simulink model "image_analysis_color"  (Simulink 7.6)
settings: Solver=FixedStepDiscrete  StartTime=0.0  StopTime=0  RelTol=1e-3
undefined symbols (not defined in the file or in its folder): Iter_Segment_Thresh, jet, Rec, SDTV
libraries: vipsnks x16, vipconversions x11, vipanalysis x4, vipgeotforms x3, viptransforms x2, vipsrcs x1, viptextngfix x1
settings Model: Creator=Administrator  LastModifiedBy=Administrator

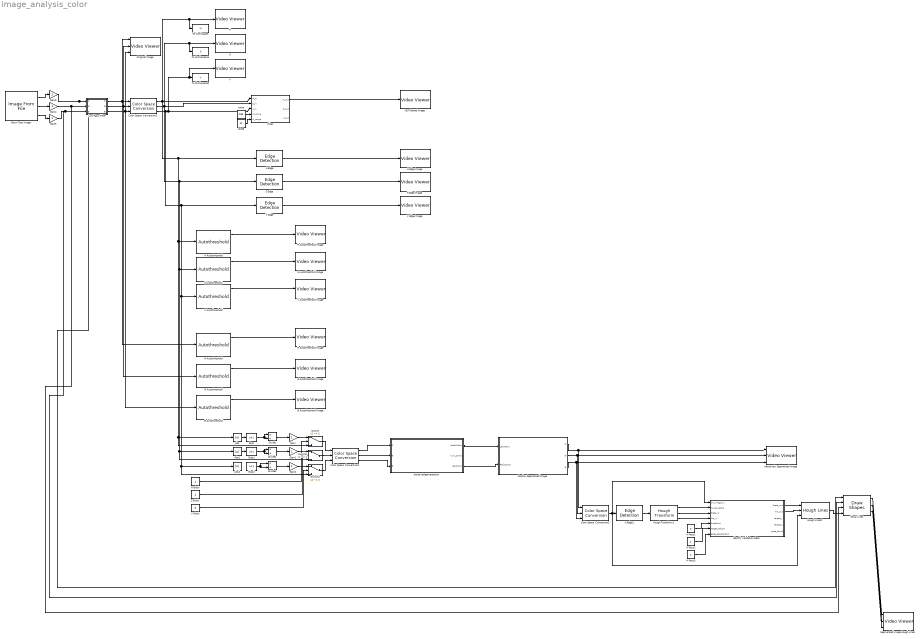
== system image_analysis_color ==
  Abs : Abs
  Abs1 : Abs
  Abs2 : Abs
  B Autothreshold : vipconversions/Autothreshold  DialogController=vipDDGCreate  DialogControllerArgs=DataTag0  operator=>  threshOut=on  effMetricOut=on  userDefinedRange=off  umin=0  umax=255  outOfRngOpt=Warn and saturate  scaleThreshold=off  scaleFactor=1  P1Mode=Specify word length  P1WordLength=32  P1FracLength=30  P2Mode=Specify word length  P2WordLength=32  P2FracLength=22  P3Mode=Specify word length  P3WordLength=32  P3FracLength=14  P4Mode=Binary point scaling  P4WordLength=32  P4FracLength=15  Q1Mode=Specify word length  Q1WordLength=32  Q1FracLength=16  EMMode=Specify word length  EMWordLength=16  EMFracLength=14  roundingMode=Floor  overflowMode=off
  B Autothreshold Image : vipsnks/Video Viewer  DialogControllerArgs=DataTag2  inputType=Obsolete7b  imagePorts=One multidimensional signal  useColorMap=off  colormapValue=jet(256)  specRange=off  minInputVal=0  maxInputVal=255  FigPos=[805 664 208 170]  AxisZoom=on  trueSizedOnce=off  OpenAtMdlStart=on
  Bias : Bias  Bias=1
  Bias1 : Bias  Bias=1
  Bias2 : Bias  Bias=1
  Color Space  Conversion1 : vipconversions/Color Space  Conversion  conversion=Obsolete  conversionActive=R'G'B' to HSV  wp_str=D65  rec=Rec. 601 (SDTV)  sys=1125/60/2:1  imagePorts=Separate color signals
  Color Space  Conversion2 : vipconversions/Color Space  Conversion  conversion=Obsolete  conversionActive=HSV to R'G'B'  wp_str=D65  rec=Rec. 601 (SDTV)  sys=1125/60/2:1  imagePorts=Separate color signals
  Color Space  Conversion3 : vipconversions/Color Space  Conversion  conversion=Obsolete  conversionActive=R'G'B' to intensity  wp_str=D65  rec=Rec. 601 (SDTV)  sys=1125/60/2:1  imagePorts=Separate color signals
  Display Segmented Image : Subsystem
      settings: UndoDeleteFcn=Stateflow.SLINSF.SimulinkMan.restorePreDeleteFcn  PreDeleteFcn=Stateflow.SLINSF.SimulinkMan.removePreDeleteFcn
  Divide : Product  Inputs=*/
  Divide1 : Product  Inputs=*/
  Divide2 : Product  Inputs=*/
  Down Test Image : vipsrcs/Image From File  Tag=vipblks_nd  DialogController=vipDDGCreate  DialogControllerArgs=DataTag3  SystemSampleTime=-1  FileName=C:\Documents and Settings\Administrator\My Documents\Academics\Summer 2011\Digital Image Correlation\Sample Pictures 5-24-11\sample1_small.JPG  imagePorts=Separate color signals  Ts=-1  ImageDataType=double  Signed=on  WordLength=16  sdImageDataType=uint(8)  FractionLengthMode=User-defined  FractionLength=15  OutPortLabels=R|G|B
  Draw Lines : viptextngfix/Draw Shapes  DialogController=vipDDGCreate  DialogControllerArgs=DataTag4  shape=Lines  fill=off  fillClrSource=Specify via dialog  display=User-specified value  intensity=200  color=[.8 .8 .8]  opacity=0.6  viewport=Entire image  antialiasing=off  inType=Obsolete  imagePorts=Separate color signals  prodOutputMode=Binary point scaling  prodOutputWordLength=32  prodOutputFracLength=14  memoryMode=Specify word length  memoryWordLength=16  memoryFracLength=15  roundingMode=Floor  overflowMode=off
  Filter : Stateflow chart  TreatAsAtomicUnit=on
  G Autothreshold : vipconversions/Autothreshold  DialogController=vipDDGCreate  DialogControllerArgs=DataTag5  operator=>  threshOut=on  effMetricOut=on  userDefinedRange=off  umin=0  umax=255  outOfRngOpt=Warn and saturate  scaleThreshold=off  scaleFactor=1  P1Mode=Specify word length  P1WordLength=32  P1FracLength=30  P2Mode=Specify word length  P2WordLength=32  P2FracLength=22  P3Mode=Specify word length  P3WordLength=32  P3FracLength=14  P4Mode=Binary point scaling  P4WordLength=32  P4FracLength=15  Q1Mode=Specify word length  Q1WordLength=32  Q1FracLength=16  EMMode=Specify word length  EMWordLength=16  EMFracLength=14  roundingMode=Floor  overflowMode=off
  G Autothreshold Image : vipsnks/Video Viewer  DialogControllerArgs=DataTag7  inputType=Obsolete7b  imagePorts=One multidimensional signal  useColorMap=off  colormapValue=jet(256)  specRange=off  minInputVal=0  maxInputVal=255  FigPos=[794 437 202 172]  AxisZoom=on  trueSizedOnce=off  OpenAtMdlStart=on
  Gain{,1..5} (6 alike) : Gain
  H : vipsnks/Video Viewer  DialogControllerArgs=DataTag9  inputType=Obsolete7b  imagePorts=One multidimensional signal  useColorMap=off  colormapValue=jet(256)  specRange=off  minInputVal=0  maxInputVal=255  FigPos=[177 241 253 152]  AxisZoom=on  trueSizedOnce=off  OpenAtMdlStart=on
  H Autothreshold : vipconversions/Autothreshold  DialogController=vipDDGCreate  DialogControllerArgs=DataTag10  operator=>  threshOut=on  effMetricOut=on  userDefinedRange=off  umin=0  umax=255  outOfRngOpt=Warn and saturate  scaleThreshold=off  scaleFactor=1  P1Mode=Specify word length  P1WordLength=32  P1FracLength=30  P2Mode=Specify word length  P2WordLength=32  P2FracLength=22  P3Mode=Specify word length  P3WordLength=32  P3FracLength=14  P4Mode=Binary point scaling  P4WordLength=32  P4FracLength=15  Q1Mode=Specify word length  Q1WordLength=32  Q1FracLength=16  EMMode=Specify word length  EMWordLength=16  EMFracLength=14  roundingMode=Floor  overflowMode=off
  H Autothreshold Image : vipsnks/Video Viewer  DialogControllerArgs=DataTag12  inputType=Obsolete7b  imagePorts=One multidimensional signal  useColorMap=off  colormapValue=jet(256)  specRange=off  minInputVal=0  maxInputVal=255  FigPos=[602 227 224 146]  AxisZoom=on  trueSizedOnce=off  OpenAtMdlStart=on
  H Block : Constant
  H Edge : vipanalysis/Edge Detection  DialogController=vipDDGCreate  DialogControllerArgs=DataTag13  method=Sobel  outputType=Binary image  userDefinedThreshold=off  thresholdSource=Specify via dialog  threshold=20  thresholdTuning=3  edgeThinning=on  threshold_canny=[0.25 0.60]  autoPercent=70  sigma=1  roundingMode=Floor  overflowMode=off
  H Edge Image : vipsnks/Video Viewer  DialogControllerArgs=DataTag15  inputType=Obsolete7b  imagePorts=One multidimensional signal  useColorMap=off  colormapValue=jet(256)  specRange=off  minInputVal=0  maxInputVal=255  FigPos=[390 221 222 140]  AxisZoom=on  trueSizedOnce=off  OpenAtMdlStart=on
  H Edge1 : vipanalysis/Edge Detection  DialogController=vipDDGCreate  DialogControllerArgs=DataTag16  method=Sobel  outputType=Binary image  userDefinedThreshold=off  thresholdSource=Specify via dialog  threshold=20  thresholdTuning=3  edgeThinning=on  threshold_canny=[0.25 0.60]  autoPercent=70  sigma=1  roundingMode=Floor  overflowMode=off
  H Pass1 : Constant  Value=0
  H Pass2 : Constant
  H Pass3 : Constant
  HS Filtered Image : vipsnks/Video Viewer  DialogControllerArgs=DataTag18  inputType=Obsolete7b  imagePorts=One multidimensional signal  useColorMap=off  colormapValue=jet(256)  specRange=off  minInputVal=0  maxInputVal=255  FigPos=[-38 479 226 177]  AxisZoom=on  trueSizedOnce=off  OpenAtMdlStart=on
  Hough Lines2 : viptransforms/Hough Lines  DialogController=vipDDGCreate  DialogControllerArgs=DataTag19  sineCompMethod=Trigonometric function  thetaRes=pi/180  firstCoeffMode=Specify word length  firstCoeffWordLength=16  firstCoeffFracLength=15  prodOutputMode=Binary point scaling  prodOutputWordLength=32  prodOutputFracLength=16  roundingMode=Nearest  overflowMode=on
  Hough Transform1 : viptransforms/Hough Transform  DialogController=vipDDGCreate  DialogControllerArgs=DataTag20  theta_res=pi/180  rho_res=1  out_theta_rho=on  outdtmode=double  firstCoeffMode=Binary point scaling  firstCoeffWordLength=16  firstCoeffFracLength=14  secondCoeffMode=Binary point scaling  secondCoeffWordLength=32  secondCoeffFracLength=16  outputMode=Binary point scaling  outputWordLength=16  outputFracLength=0  accumMode=Binary point scaling  accumWordLength=32  accumFracLength=20  prodOutputMode=Binary point scaling  prodOutputWordLength=32  prodOutputFracLength=20  memoryMode=Binary point scaling  memoryWordLength=32  memoryFracLength=16  roundingMode=Nearest  overflowMode=on
  Identify Validation Gate : Stateflow chart  TreatAsAtomicUnit=on  SystemSampleTime=[1/30 0]
  IterativeSegmentation : Subsystem
      settings: UndoDeleteFcn=Stateflow.SLINSF.SimulinkMan.restorePreDeleteFcn  PreDeleteFcn=Stateflow.SLINSF.SimulinkMan.removePreDeleteFcn
  Iteratively Segmented Image : vipsnks/Video Viewer  DialogControllerArgs=DataTag25  inputType=Obsolete7b  imagePorts=Separate color signals  useColorMap=off  colormapValue=jet(256)  specRange=off  minInputVal=0  maxInputVal=255  FigPos=[1060 242 237 156]  AxisZoom=on  trueSizedOnce=off  OpenAtMdlStart=on
  Low Pass Filter : Subsystem
  Original Image : vipsnks/Video Viewer  DialogControllerArgs=DataTag27  inputType=Obsolete7b  imagePorts=Separate color signals  useColorMap=off  colormapValue=jet(256)  specRange=off  minInputVal=0  maxInputVal=255  FigPos=[-27 258 221 180]  AxisZoom=on  trueSizedOnce=off  OpenAtMdlStart=on
  R Autothreshold : vipconversions/Autothreshold  DialogController=vipDDGCreate  DialogControllerArgs=DataTag28  operator=>  threshOut=on  effMetricOut=on  userDefinedRange=off  umin=0  umax=255  outOfRngOpt=Warn and saturate  scaleThreshold=off  scaleFactor=1  P1Mode=Specify word length  P1WordLength=32  P1FracLength=30  P2Mode=Specify word length  P2WordLength=32  P2FracLength=22  P3Mode=Specify word length  P3WordLength=32  P3FracLength=14  P4Mode=Binary point scaling  P4WordLength=32  P4FracLength=15  Q1Mode=Specify word length  Q1WordLength=32  Q1FracLength=16  EMMode=Specify word length  EMWordLength=16  EMFracLength=14  roundingMode=Floor  overflowMode=off
  R Autothreshold Image : vipsnks/Video Viewer  DialogControllerArgs=DataTag30  inputType=Obsolete7b  imagePorts=One multidimensional signal  useColorMap=off  colormapValue=jet(256)  specRange=off  minInputVal=0  maxInputVal=255  FigPos=[794 238 224 156]  AxisZoom=on  trueSizedOnce=off  OpenAtMdlStart=on
  S : vipsnks/Video Viewer  DialogControllerArgs=DataTag32  inputType=Obsolete7b  imagePorts=One multidimensional signal  useColorMap=off  colormapValue=jet(256)  specRange=off  minInputVal=0  maxInputVal=255  FigPos=[193 436 207 154]  AxisZoom=on  trueSizedOnce=off  OpenAtMdlStart=on
  S Autothreshold : vipconversions/Autothreshold  DialogController=vipDDGCreate  DialogControllerArgs=DataTag33  operator=>  threshOut=on  effMetricOut=on  userDefinedRange=off  umin=0  umax=255  outOfRngOpt=Warn and saturate  scaleThreshold=off  scaleFactor=1  P1Mode=Specify word length  P1WordLength=32  P1FracLength=30  P2Mode=Specify word length  P2WordLength=32  P2FracLength=22  P3Mode=Specify word length  P3WordLength=32  P3FracLength=14  P4Mode=Binary point scaling  P4WordLength=32  P4FracLength=15  Q1Mode=Specify word length  Q1WordLength=32  Q1FracLength=16  EMMode=Specify word length  EMWordLength=16  EMFracLength=14  roundingMode=Floor  overflowMode=off
  S Autothreshold Image : vipsnks/Video Viewer  DialogControllerArgs=DataTag35  inputType=Obsolete7b  imagePorts=One multidimensional signal  useColorMap=off  colormapValue=jet(256)  specRange=off  minInputVal=0  maxInputVal=255  FigPos=[572 439 254 167]  AxisZoom=on  trueSizedOnce=off  OpenAtMdlStart=on
  S Block : Constant
  S Edge : vipanalysis/Edge Detection  DialogController=vipDDGCreate  DialogControllerArgs=DataTag36  method=Sobel  outputType=Binary image  userDefinedThreshold=off  thresholdSource=Specify via dialog  threshold=20  thresholdTuning=3  edgeThinning=on  threshold_canny=[0.25 0.60]  autoPercent=70  sigma=1  roundingMode=Floor  overflowMode=off
  S Edge Image : vipsnks/Video Viewer  DialogControllerArgs=DataTag38  inputType=Obsolete7b  imagePorts=One multidimensional signal  useColorMap=off  colormapValue=jet(256)  specRange=off  minInputVal=0  maxInputVal=255  FigPos=[396 426 193 132]  AxisZoom=on  trueSizedOnce=off  OpenAtMdlStart=on
  Segmented Image Hough Lines : vipsnks/Video Viewer  DialogControllerArgs=DataTag40  inputType=Obsolete7b  imagePorts=Separate color signals  useColorMap=off  colormapValue=jet(256)  specRange=off  minInputVal=0  maxInputVal=255  FigPos=[1009 491 272 162]  AxisZoom=on  trueSizedOnce=off  OpenAtMdlStart=on
  Switch : Switch  Criteria=u2 ~= 0
  Switch1 : Switch  Criteria=u2 ~= 0
  Switch2 : Switch  Criteria=u2 ~= 0
  To Workspace : ToWorkspace  VariableName=H  SampleTime=-1  SaveFormat=Array
  To Workspace1 : ToWorkspace  VariableName=S  SampleTime=-1  SaveFormat=Array
  To Workspace2 : ToWorkspace  VariableName=V  SampleTime=-1  SaveFormat=Array
  V : vipsnks/Video Viewer  DialogControllerArgs=DataTag42  inputType=Obsolete7b  imagePorts=One multidimensional signal  useColorMap=off  colormapValue=jet(256)  specRange=off  minInputVal=0  maxInputVal=255  FigPos=[202 649 196 150]  AxisZoom=on  trueSizedOnce=off  OpenAtMdlStart=on
  V Autothreshold : vipconversions/Autothreshold  DialogController=vipDDGCreate  DialogControllerArgs=DataTag43  operator=>  threshOut=on  effMetricOut=on  userDefinedRange=off  umin=0  umax=255  outOfRngOpt=Warn and saturate  scaleThreshold=off  scaleFactor=1  P1Mode=Specify word length  P1WordLength=32  P1FracLength=30  P2Mode=Specify word length  P2WordLength=32  P2FracLength=22  P3Mode=Specify word length  P3WordLength=32  P3FracLength=14  P4Mode=Binary point scaling  P4WordLength=32  P4FracLength=15  Q1Mode=Specify word length  Q1WordLength=32  Q1FracLength=16  EMMode=Specify word length  EMWordLength=16  EMFracLength=14  roundingMode=Floor  overflowMode=off
  V Autothreshold Image : vipsnks/Video Viewer  DialogControllerArgs=DataTag45  inputType=Obsolete7b  imagePorts=One multidimensional signal  useColorMap=off  colormapValue=jet(256)  specRange=off  minInputVal=0  maxInputVal=255  FigPos=[556 659 250 172]  AxisZoom=on  trueSizedOnce=off  OpenAtMdlStart=on
  V Block : Constant  Value=0
  V Edge : vipanalysis/Edge Detection  DialogController=vipDDGCreate  DialogControllerArgs=DataTag46  method=Sobel  outputType=Binary image  userDefinedThreshold=off  thresholdSource=Specify via dialog  threshold=20  thresholdTuning=3  edgeThinning=on  threshold_canny=[0.25 0.60]  autoPercent=70  sigma=1  roundingMode=Floor  overflowMode=off
  V Edge Image : vipsnks/Video Viewer  DialogControllerArgs=DataTag48  inputType=Obsolete7b  imagePorts=One multidimensional signal  useColorMap=off  colormapValue=jet(256)  specRange=off  minInputVal=0  maxInputVal=255  FigPos=[381 650 208 142]  AxisZoom=on  trueSizedOnce=off  OpenAtMdlStart=on
  range : Constant  Value=.11  SampleTime=-1
  value : Constant  Value=.195  SampleTime=-1
  wires:
  Color Space  Conversion1/1 -> Filter/1(H_in), H/1, To Workspace/1, H Edge/1, H Autothreshold/1, Switch/3, Abs/1
  Color Space  Conversion1/2 -> Filter/2(S_in), S/1, To Workspace1/1, S Edge/1, S Autothreshold/1, Switch1/3, Abs1/1
  Filter/1(H_out) -> HS Filtered Image/1
  value/1 -> Filter/4(H_value)
  range/1 -> Filter/5(H_range)
  Color Space  Conversion1/3 -> V/1, To Workspace2/1, Filter/3(V_in), V Edge/1, V Autothreshold/1, Switch2/3, Abs2/1
  H Edge/1 -> H Edge Image/1
  S Edge/1 -> S Edge Image/1
  V Edge/1 -> V Edge Image/1
  Down Test Image/2 -> Gain4/1
  Down Test Image/1 -> Gain3/1
  Down Test Image/3 -> Gain5/1
  Low Pass Filter/2(G') -> Color Space  Conversion1/2, Original Image/2, G Autothreshold/1
  Low Pass Filter/3(B') -> Color Space  Conversion1/3, Original Image/3, B Autothreshold/1
  Low Pass Filter/1(R') -> Color Space  Conversion1/1, Original Image/1, R Autothreshold/1
  Display Segmented Image/1(R) -> Color Space  Conversion3/1, Iteratively Segmented Image/1
  Display Segmented Image/2(G) -> Color Space  Conversion3/2, Iteratively Segmented Image/2
  Display Segmented Image/3(B) -> Color Space  Conversion3/3, Iteratively Segmented Image/3
  IterativeSegmentation/1(LabelMatrix) -> Display Segmented Image/1(LabMatrix)
  IterativeSegmentation/3(ref_colors) -> Display Segmented Image/2(Ref_Colors)
  H Autothreshold/1 -> H Autothreshold Image/1
  S Autothreshold/1 -> S Autothreshold Image/1
  V Autothreshold/1 -> V Autothreshold Image/1
  R Autothreshold/1 -> R Autothreshold Image/1
  G Autothreshold/1 -> G Autothreshold Image/1
  B Autothreshold/1 -> B Autothreshold Image/1
  Color Space  Conversion2/3 -> IterativeSegmentation/3(B)
  Color Space  Conversion2/2 -> IterativeSegmentation/2(G)
  Color Space  Conversion2/1 -> IterativeSegmentation/1(R)
  Divide/1 -> Gain/1
  Abs/1 -> Bias/1
  Bias/1 -> Divide/1, Divide/2
  Divide1/1 -> Gain1/1
  Abs1/1 -> Bias1/1
  Bias1/1 -> Divide1/1, Divide1/2
  Switch1/1 -> Color Space  Conversion2/2
  Switch/1 -> Color Space  Conversion2/1
  Switch2/1 -> Color Space  Conversion2/3
  Bias2/1 -> Divide2/1, Divide2/2
  Gain/1 -> Switch/1
  Gain1/1 -> Switch1/1
  Gain2/1 -> Switch2/1
  Divide2/1 -> Gain2/1
  H Block/1 -> Switch/2
  S Block/1 -> Switch1/2
  V Block/1 -> Switch2/2
  Color Space  Conversion3/1 -> Hough Lines2/3, H Edge1/1, Identify Validation Gate/1(bw_image_in)
  Hough Transform1/1 -> Identify Validation Gate/2(hough_table)
  Hough Transform1/2 -> Identify Validation Gate/3(theta_in)
  Hough Transform1/3 -> Identify Validation Gate/4(rho_in)
  H Pass1/1 -> Identify Validation Gate/5(threshold)
  H Pass2/1 -> Identify Validation Gate/6(target_height)
  H Pass3/1 -> Identify Validation Gate/7(gate_aspect_ratio)
  Identify Validation Gate/1(theta_out) -> Hough Lines2/1
  Identify Validation Gate/2(rho_out) -> Hough Lines2/2
  H Edge1/1 -> Hough Transform1/1
  Hough Lines2/1 -> Draw Lines/4
  Draw Lines/1 -> Segmented Image Hough Lines/1
  Draw Lines/2 -> Segmented Image Hough Lines/2
  Draw Lines/3 -> Segmented Image Hough Lines/3
  Gain3/1 -> Low Pass Filter/1(R), Draw Lines/1
  Gain4/1 -> Low Pass Filter/2(G), Draw Lines/3
  Gain5/1 -> Low Pass Filter/3(B), Draw Lines/2

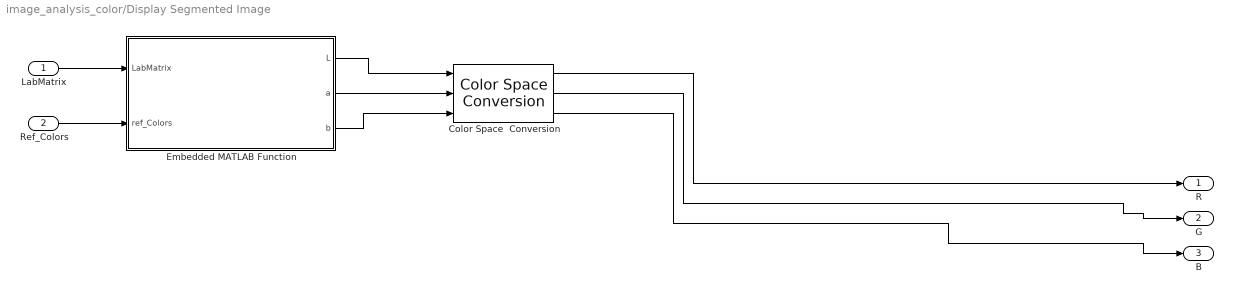
== system image_analysis_color/Display Segmented Image ==
  LabMatrix : Inport
  Ref_Colors : Inport  Port=2
  Color Space  Conversion : vipconversions/Color Space  Conversion  conversion=Obsolete  conversionActive=L*a*b* to sR'G'B'  wp_str=D50  rec=Rec. 601 (SDTV)  sys=1125/60/2:1  imagePorts=Separate color signals
  Embedded MATLAB Function : Stateflow chart  TreatAsAtomicUnit=on
  R : Outport  OutDataTypeStr=double
  G : Outport  Port=2  OutDataTypeStr=double
  B : Outport  Port=3  OutDataTypeStr=double
  wires:
  Color Space  Conversion/3 -> B/1
  Color Space  Conversion/2 -> G/1
  Color Space  Conversion/1 -> R/1
  Embedded MATLAB Function/3(b) -> Color Space  Conversion/3
  Embedded MATLAB Function/2(a) -> Color Space  Conversion/2
  Embedded MATLAB Function/1(L) -> Color Space  Conversion/1
  Ref_Colors/1 -> Embedded MATLAB Function/2(ref_Colors)
  LabMatrix/1 -> Embedded MATLAB Function/1(LabMatrix)

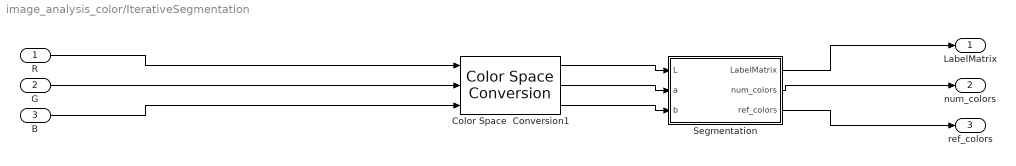
== system image_analysis_color/IterativeSegmentation ==
  R : Inport
  G : Inport  Port=2
  B : Inport  Port=3
  Color Space  Conversion1 : vipconversions/Color Space  Conversion  conversion=Obsolete  conversionActive=sR'G'B' to L*a*b*  wp_str=D50  rec=Rec. 601 (SDTV)  sys=1125/60/2:1  imagePorts=Separate color signals
  Segmentation : Subsystem
  LabelMatrix : Outport
  num_colors : Outport  Port=2
  ref_colors : Outport  Port=3
  wires:
  Segmentation/3(ref_colors) -> ref_colors/1
  Segmentation/2(num_colors) -> num_colors/1
  Segmentation/1(LabelMatrix) -> LabelMatrix/1
  Color Space  Conversion1/3 -> Segmentation/3(b)
  Color Space  Conversion1/2 -> Segmentation/2(a)
  Color Space  Conversion1/1 -> Segmentation/1(L)
  R/1 -> Color Space  Conversion1/1
  G/1 -> Color Space  Conversion1/2
  B/1 -> Color Space  Conversion1/3

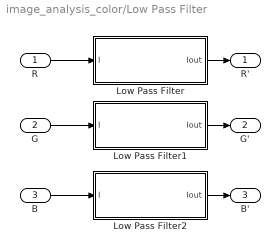
== system image_analysis_color/Low Pass Filter ==
  R : Inport
  G : Inport  Port=2
  B : Inport  Port=3
  Low Pass Filter : Stateflow chart  TreatAsAtomicUnit=on
  Low Pass Filter1 : Stateflow chart  TreatAsAtomicUnit=on
  Low Pass Filter2 : Stateflow chart  TreatAsAtomicUnit=on
  R' : Outport
  G' : Outport  Port=2
  B' : Outport  Port=3
  wires:
  Low Pass Filter/1(Iout) -> R'/1
  Low Pass Filter2/1(Iout) -> B'/1
  Low Pass Filter1/1(Iout) -> G'/1
  B/1 -> Low Pass Filter2/1(I)
  G/1 -> Low Pass Filter1/1(I)
  R/1 -> Low Pass Filter/1(I)

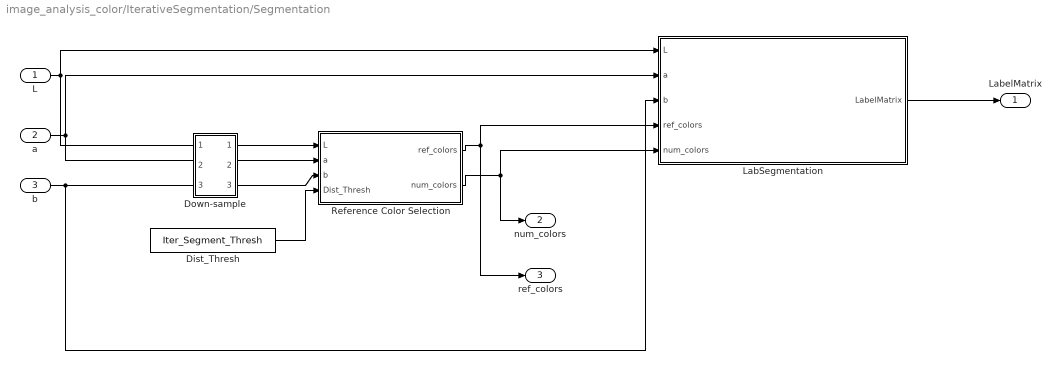
== system image_analysis_color/IterativeSegmentation/Segmentation ==
  L : Inport
  a : Inport  Port=2
  b : Inport  Port=3
  Dist_Thresh : Constant  Value=Iter_Segment_Thresh  SampleTime=-1
  Down-sample : Subsystem
  LabSegmentation : Stateflow chart  TreatAsAtomicUnit=on
  Reference Color Selection : Stateflow chart  TreatAsAtomicUnit=on
  LabelMatrix : Outport
  num_colors : Outport  Port=2
  ref_colors : Outport  Port=3
  wires:
  Dist_Thresh/1 -> Reference Color Selection/4(Dist_Thresh)
  LabSegmentation/1(LabelMatrix) -> LabelMatrix/1
  Reference Color Selection/2(num_colors) -> LabSegmentation/5(num_colors), num_colors/1
  Reference Color Selection/1(ref_colors) -> ref_colors/1, LabSegmentation/4(ref_colors)
  b/1 -> LabSegmentation/3(b), Reference Color Selection/3(b)
  a/1 -> LabSegmentation/2(a), Reference Color Selection/2(a)
  L/1 -> LabSegmentation/1(L), Reference Color Selection/1(L)

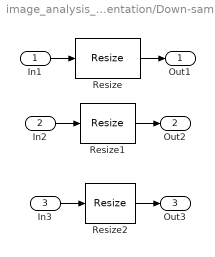
== system image_analysis_color/IterativeSegmentation/Segmentation/Down-sample ==
  In1 : Inport
  In2 : Inport  Port=2
  In3 : Inport  Port=3
  Resize : vipgeotforms/Resize  DialogController=vipDDGCreate  DialogControllerArgs=DataTag21  specify=Number of output rows and columns  rfactor=[]  outCols=25  outRows=25  outRowsCols=[60 80]  interp_method=Bilinear  antialias=on  useROI=off  roiFlag=off  prodOutputMode=Binary point scaling  prodOutputWordLength=32  prodOutputFracLength=10  roundingMode=Nearest  overflowMode=on
  Resize1 : vipgeotforms/Resize  DialogController=vipDDGCreate  DialogControllerArgs=DataTag22  specify=Number of output rows and columns  rfactor=[200 150]  outCols=25  outRows=25  outRowsCols=[60 80]  interp_method=Bilinear  antialias=on  useROI=off  roiFlag=off  prodOutputMode=Binary point scaling  prodOutputWordLength=32  prodOutputFracLength=10  roundingMode=Nearest  overflowMode=on
  Resize2 : vipgeotforms/Resize  DialogController=vipDDGCreate  DialogControllerArgs=DataTag23  specify=Number of output rows and columns  rfactor=[200 150]  outCols=25  outRows=25  outRowsCols=[60 80]  interp_method=Bilinear  antialias=on  useROI=off  roiFlag=off  prodOutputMode=Binary point scaling  prodOutputWordLength=32  prodOutputFracLength=10  roundingMode=Nearest  overflowMode=on
  Out1 : Outport
  Out2 : Outport  Port=2
  Out3 : Outport  Port=3
  wires:
  Resize2/1 -> Out3/1
  In3/1 -> Resize2/1
  Resize1/1 -> Out2/1
  In2/1 -> Resize1/1
  Resize/1 -> Out1/1
  In1/1 -> Resize/1

== matlab function Display Segmented Image/Embedded MATLAB Function ==
  data: LabMatrix input double; L output double; ref_Colors input double; a output double; b output double
function [L,a,b]=CombineSegmentedImage(LabMatrix,ref_Colors)
% This function puts together the segmented imaged such that it can be shown

[rows, cols] = size(LabMatrix);
L = zeros(rows,cols);
a = zeros(rows,cols);
b = zeros(rows,cols);

for i = 1:rows
    for j = 1:cols
        L(i,j) = ref_Colors(LabMatrix(i,j),1);
        a(i,j) = ref_Colors(LabMatrix(i,j),2);
        b(i,j) = ref_Colors(LabMatrix(i,j),3);
    end
end

return

== matlab function Identify Validation Gate ==
  data: bw_image_in input double; hough_table input double; theta_out output double; rho_out output double; target_y output double; target_z output double; gate_found output double; theta_in input double; rho_in input double; threshold input double; target_height input double; gate_aspect_ratio input double
function [theta_out, rho_out, target_y, target_z, gate_found] = validation_gate(bw_image_in, hough_table, theta_in, rho_in, threshold, target_height, gate_aspect_ratio)
%#eml

% This function attempts to identfiy the validation gate, and returns line
%   information, targeting information, and a true/false gate_found
%   parameter.
%
% 5-29-11
%
% Input
%
%   target_height = fraction of goal post height to aim AUV at
%   gate_aspect_ratio = used to infer unknown points with little extra
%     processing (height/width of large T-shape)
%
% Output
%
% Notes:
%   The hough_table is destroyed in this function (acceptable if
%     hough_table is not an output)
%   Process:
%     1. Identify primary, relatively "long" lines
%     2. 

% Initialize
peak_tol_ratio = .1;  % Fraction of max(rows,cols) of image within which a
%                         peak is assumed to reside; this helps reduce
%                         incorrect line extraction
max_num_lines = 20;  % Considers this many popular lines as candidates

[rho_length, theta_length] = size(hough_table);
[rows, cols] = size(bw_image_in);
rho_tol = .1*max(rows,cols);
theta_tol = 10*pi/180;  % Tolerence within which two slopes are equal (radians)

rho = zeros(1,max_num_lines);
theta = zeros(1,max_num_lines);
rho_out = rho;
theta_out = theta;
%rho_out = zeros(1,3);
%theta_out = zeros(1,3);



% Apply appropriate threshold
hough_table = hough_table.*( hough_table >= threshold );


% Identify the most likely max_num_lines lines
i_index = ones(1,max_num_lines);
j_index = ones(1,max_num_lines);

m = 1;
while( m <= max_num_lines )
    
    max_votes = 0;
    for i = 1:rho_length
        for j = 1:theta_length
            if( hough_table(i,j) > max_votes )
                i_index(m) = i;
                j_index(m) = j;
                max_votes = hough_table(i,j);
            end
        end
    end
    
    rho(m) = rho_in(i_index(m));
    theta(m) = theta_in(j_index(m));
    hough_table(i_index(m),j_index(m)) = 0;
    m = m + 1;
    
end


% Extract the three most popular lines that fit the geometric criteria for
%   the goalpost
rho_out(1) = rho(1);
theta_out(1) = theta(1);

m = 2;

%rho_radius = 10;
%theta_radius = 5*pi/180;

for i = 2:max_num_lines
    
    % If rho, theta do not match within tolerance, then store as the next
    %   line
%    if( ( (rho(m) - rho(1))/rho_radius)^2 + ( (theta(m) - theta(1))/theta_radius)^2 > 1 )
    if( abs(rho(i) - rho(i-1)) >= 30 )
        rho_out(m) = rho(i);
        theta_out(m) = theta(i);
        m = m + 1;
        if( m > 3 )
            break;
        end
    end
    
end


% Determine whether or not the top three lines constitute the goal post
%   Note that the Simulink block feeding this function keeps theta between
%   +/- pi/2
if( abs(theta_out(1) - theta_out(2)) < theta_tol && ( max(theta_out(1),theta_out(3)) - min(theta_out(1),theta_out(3)) - pi/2 < theta_tol ) )
    gate_found = 1;
    avg_slope = -( 1/tan(theta_out(1)) + 1/tan(theta_out(2)) )/2;
    y1 = ( (rho_out(1)/cos(theta_out(1))) - (rho_out(3)/cos(theta_out(3))) )*( 1/( tan(theta_out(1)) - tan(theta_out(3)) ) );
    x1 = ( 1/cos(theta_out(1)) )*( rho_out(1) - y1*sin(theta_out(1)) );
    y2 = ( (rho_out(2)/cos(theta_out(2))) - (rho_out(3)/cos(theta_out(3))) )*( 1/( tan(theta_out(2)) - tan(theta_out(3)) ) );
    x2 = ( 1/cos(theta_out(2)) )*( rho_out(2) - y2*sin(theta_out(2)) );
    
elseif( abs(theta_out(1) - theta_out(3)) < theta_tol && ( max(theta_out(1),theta_out(2)) - min(theta_out(1),theta_out(2)) - pi/2 < theta_tol ) )
    gate_found = 1;
    avg_slope = -( 1/tan(theta_out(1)) + 1/tan(theta_out(3)) )/2;
    y1 = ( (rho_out(1)/cos(theta_out(1))) - (rho_out(2)/cos(theta_out(2))) )*( 1/( tan(theta_out(1)) - tan(theta_out(2)) ) );
    x1 = ( 1/cos(theta_out(1)) )*( rho_out(1) - y1*sin(theta_out(1)) );
    y2 = ( (rho_out(2)/cos(theta_out(2))) - (rho_out(3)/cos(theta_out(3))) )*( 1/( tan(theta_out(2)) - tan(theta_out(3)) ) );
    x2 = ( 1/cos(theta_out(2)) )*( rho_out(2) - y2*sin(theta_out(2)) );
    
elseif( abs(theta_out(2) - theta_out(3)) < theta_tol && ( max(theta_out(1),theta_out(2)) - min(theta_out(1),theta_out(2)) - pi/2 < theta_tol ) )
    gate_found = 1;
    avg_slope = -( 1/tan(theta_out(2)) + 1/tan(theta_out(3)) )/2;
    y1 = ( (rho_out(1)/cos(theta_out(1))) - (rho_out(2)/cos(theta_out(2))) )*( 1/( tan(theta_out(1)) - tan(theta_out(2)) ) );
    x1 = ( 1/cos(theta_out(1)) )*( rho_out(1) - y1*sin(theta_out(1)) );
    y2 = ( (rho_out(1)/cos(theta_out(1))) - (rho_out(3)/cos(theta_out(3))) )*( 1/( tan(theta_out(1)) - tan(theta_out(3)) ) );
    x2 = ( 1/cos(theta_out(1)) )*( rho_out(1) - y2*sin(theta_out(1)) );
    
else
    gate_found = 0;
    avg_slope = 0;
    
    x1 = 0;
    y1 = 0;
    x2 = 0;
    y2 = 0;
    
end


% Determine targeting information (default to center of viewing area if no
%   gate found)
if( gate_found ~= 0 )
    
    % Determine width and half-height (to center of goal post)
    w = sqrt( (x2 - x1)^2 + (y2 - y1)^2 );
    hh = target_height*gate_aspect_ratio*w;
    
    % Project a line "up" (relative to camera) and determine target
    %   information
    x12 = (x1 + x2)/2;
    y12 = (y1 + y2)/2;
    
    u = [1 -abs(avg_slope)];
    u = u./norm(u);
    
    target_x = x12 + hh*u(1);
    target_y = y12 + hh*u(2);
    
    
    % old code that works, partially
    %phi = atan(avg_slope);
    %target_x = x12 - hh*cos(phi);
    %target_y = y12 - hh*sin(phi);
    
    
    
    
    
    
    %{
    intercept = y12 - avg_slope*x12;
    
    a = avg_slope^2 + 1;
    b = 2*(avg_slope*(intercept - y12) - x12);
    c = x12^2 + (avg_slope - y12)^2 - hh^2;
    
    target_x = real( (-b + sqrt(b^2 - 4*a*c))/(2*a) );
    target_y = avg_slope*target_x + intercept;
    %}
    
    
    
    % Transform target x, y to global coordinate system
    target_z = target_y - floor(rows/2);
    target_y = target_x - floor(cols/2);
    
else
    
    % Default is center of viewing area
    target_x = 0;
    target_y = 0;
    target_z = 0;
    
end



%%debub
rho_out = rho;
theta_out = theta;
%%/debug



return

== matlab function Filter ==
  data: H_in input double; S_in input double; V_in input double; H_value input double; H_range input double; H_out output double; S_out output double; V_out output double
function [H_out, S_out, V_out] = test_filter(H_in, S_in, V_in, H_value, H_range)  %H_lower, H_upper)
% This function extracts the pixels containing hues that path elements are
%   expected to have


% Initialize
H_out = double(H_in);
S_out = double(S_in);

H_lower = H_value - H_range/2;
H_upper = H_value + H_range/2;


% Set values outside valid ranges to zero
for i = 1:size(H_in,1)
    for j = 1:size(H_in,2)
        
        if( H_in(i,j) >= H_lower && H_in(i,j) <= H_upper )
            H_out(i,j) = 1;
        else
            H_out(i,j) = 0;
        end
        
    end
end



V_out = double(V_in);

return

== matlab function Low Pass Filter/Low Pass Filter ==
  data: I input double; Iout output double
function Iout = GaussianBlurr(I)
% This function calculates the gaussian blur of an intensity image

sigma = sqrt(2);

Grows = 3;    % Gaussian matrix rows
Gcols = 3;    % Gaussian matrix columns

[Irows Icols] = size(I);

Iout = double(zeros(Irows,Icols));

Trows = Irows - Grows + 1;
Tcols = Icols - Gcols + 1;
Itemp = double(zeros(Trows,Tcols));

G = zeros(Grows,Gcols);

FirstRow = ceil(-Grows/2);
LastRow = floor(Grows/2);
FirstCol = ceil(-Gcols/2);
LastCol = floor(Gcols/2);
Gsum = 0;
for i=FirstRow:LastRow
    for j = FirstCol:LastCol
        G(i-FirstRow+1,j-FirstCol+1) = exp(-(j*j+i*i)/(2*sigma*sigma));
        Gsum = Gsum + G(i-FirstRow+1,j-FirstCol+1);
    end
end

G = G./Gsum;

Itemp = conv2(double(I),double(G),'valid');

% reflect boundaries to keep image the same size
% top
Iout((1:LastRow),(LastCol+1:Icols-LastCol)) = Itemp((1:LastRow),(1:Tcols));
% bottom
Iout((Irows-LastRow+1:Irows),(LastCol+1:Icols-LastCol)) = Itemp((Trows-LastRow+1:Trows),(1:Tcols));
% left
Iout((1+LastRow:Irows-LastRow),(1:LastCol)) = Itemp((1:Trows),(1:LastCol));
% right
Iout((1+LastRow:Irows-LastRow),(Icols-LastCol+1:Icols)) = Itemp((1:Trows),(Tcols-LastCol+1:Tcols));
% center
Iout((1+LastRow:Irows-LastRow),(1+LastCol:Icols-LastCol)) = Itemp;
% top left corner
Iout(1:LastRow,1:LastCol) = Itemp(1:LastRow,1:LastCol);
% top right corner
Iout(1:LastRow,Icols-LastCol:Icols) = Itemp(1:LastRow,Tcols-LastCol:Tcols);
% bottom left corner
Iout(Irows-LastRow:Irows,1:LastCol) = Itemp(Trows-LastRow:Trows,1:LastCol);
% bottom right corner
Iout(Irows-LastRow:Irows,Icols-LastCol:Icols) = Itemp(Trows-LastRow:Trows,Tcols-LastCol:Tcols);

return

== matlab function Low Pass Filter/Low Pass Filter1 ==
  data: I input double; Iout output double
function Iout = GaussianBlurr(I)
% This function calculates the gaussian blur of an intensity image

sigma = sqrt(2);

Grows = 3;    % Gaussian matrix rows
Gcols = 3;    % Gaussian matrix columns

[Irows Icols] = size(I);

Iout = double(zeros(Irows,Icols));

Trows = Irows - Grows + 1;
Tcols = Icols - Gcols + 1;
Itemp = double(zeros(Trows,Tcols));

G = zeros(Grows,Gcols);

FirstRow = ceil(-Grows/2);
LastRow = floor(Grows/2);
FirstCol = ceil(-Gcols/2);
LastCol = floor(Gcols/2);
Gsum = 0;
for i=FirstRow:LastRow
    for j = FirstCol:LastCol
        G(i-FirstRow+1,j-FirstCol+1) = exp(-(j*j+i*i)/(2*sigma*sigma));
        Gsum = Gsum + G(i-FirstRow+1,j-FirstCol+1);
    end
end

G = G./Gsum;

Itemp = conv2(double(I),double(G),'valid');

% reflect boundaries to keep image the same size
% top
Iout((1:LastRow),(LastCol+1:Icols-LastCol)) = Itemp((1:LastRow),(1:Tcols));
% bottom
Iout((Irows-LastRow+1:Irows),(LastCol+1:Icols-LastCol)) = Itemp((Trows-LastRow+1:Trows),(1:Tcols));
% left
Iout((1+LastRow:Irows-LastRow),(1:LastCol)) = Itemp((1:Trows),(1:LastCol));
% right
Iout((1+LastRow:Irows-LastRow),(Icols-LastCol+1:Icols)) = Itemp((1:Trows),(Tcols-LastCol+1:Tcols));
% center
Iout((1+LastRow:Irows-LastRow),(1+LastCol:Icols-LastCol)) = Itemp;
% top left corner
Iout(1:LastRow,1:LastCol) = Itemp(1:LastRow,1:LastCol);
% top right corner
Iout(1:LastRow,Icols-LastCol:Icols) = Itemp(1:LastRow,Tcols-LastCol:Tcols);
% bottom left corner
Iout(Irows-LastRow:Irows,1:LastCol) = Itemp(Trows-LastRow:Trows,1:LastCol);
% bottom right corner
Iout(Irows-LastRow:Irows,Icols-LastCol:Icols) = Itemp(Trows-LastRow:Trows,Tcols-LastCol:Tcols);

return

== matlab function Low Pass Filter/Low Pass Filter2 ==
  data: I input double; Iout output double
function Iout = GaussianBlurr(I)
% This function calculates the gaussian blur of an intensity image

sigma = sqrt(2);

Grows = 3;    % Gaussian matrix rows
Gcols = 3;    % Gaussian matrix columns

[Irows Icols] = size(I);

Iout = double(zeros(Irows,Icols));

Trows = Irows - Grows + 1;
Tcols = Icols - Gcols + 1;
Itemp = double(zeros(Trows,Tcols));

G = zeros(Grows,Gcols);

FirstRow = ceil(-Grows/2);
LastRow = floor(Grows/2);
FirstCol = ceil(-Gcols/2);
LastCol = floor(Gcols/2);
Gsum = 0;
for i=FirstRow:LastRow
    for j = FirstCol:LastCol
        G(i-FirstRow+1,j-FirstCol+1) = exp(-(j*j+i*i)/(2*sigma*sigma));
        Gsum = Gsum + G(i-FirstRow+1,j-FirstCol+1);
    end
end

G = G./Gsum;

Itemp = conv2(double(I),double(G),'valid');

% reflect boundaries to keep image the same size
% top
Iout((1:LastRow),(LastCol+1:Icols-LastCol)) = Itemp((1:LastRow),(1:Tcols));
% bottom
Iout((Irows-LastRow+1:Irows),(LastCol+1:Icols-LastCol)) = Itemp((Trows-LastRow+1:Trows),(1:Tcols));
% left
Iout((1+LastRow:Irows-LastRow),(1:LastCol)) = Itemp((1:Trows),(1:LastCol));
% right
Iout((1+LastRow:Irows-LastRow),(Icols-LastCol+1:Icols)) = Itemp((1:Trows),(Tcols-LastCol+1:Tcols));
% center
Iout((1+LastRow:Irows-LastRow),(1+LastCol:Icols-LastCol)) = Itemp;
% top left corner
Iout(1:LastRow,1:LastCol) = Itemp(1:LastRow,1:LastCol);
% top right corner
Iout(1:LastRow,Icols-LastCol:Icols) = Itemp(1:LastRow,Tcols-LastCol:Tcols);
% bottom left corner
Iout(Irows-LastRow:Irows,1:LastCol) = Itemp(Trows-LastRow:Trows,1:LastCol);
% bottom right corner
Iout(Irows-LastRow:Irows,Icols-LastCol:Icols) = Itemp(Trows-LastRow:Trows,Tcols-LastCol:Tcols);

return

== matlab function IterativeSegmentation/Segmentation/LabSegmentation ==
  data: L input double; LabelMatrix output double; a input double; b input double; ref_colors input double; num_colors input double
function LabelMatrix  = LabSegmentation(L,a,b,ref_colors,num_colors)
% This function generates the label matrix

[rows cols] = size(L);

Lout = zeros(rows,cols);
aout = zeros(rows,cols);
bout = zeros(rows,cols);

LabelMatrix = zeros(rows,cols);

for i = 1:rows
    for j = 1:cols
        min_dist = 1000;
        index = 1;
        for k = 1:num_colors
            dist = sqrt((ref_colors(k,1) - L(i,j))^2 + (ref_colors(k,2) - a(i,j))^2 + (ref_colors(k,3) - b(i,j))^2);
            if(dist < min_dist)
                min_dist = double(dist);
                index = k;
            end
        end
        LabelMatrix(i,j) = index;
    end
end

for i = 1:rows
    for j = 1:cols
        Lout(i,j) = ref_colors(LabelMatrix(i,j),1);
        aout(i,j) = ref_colors(LabelMatrix(i,j),2);
        bout(i,j) = ref_colors(LabelMatrix(i,j),3);
    end
end

cow = 1;

return

== matlab function IterativeSegmentation/Segmentation/Reference Color Selection ==
  data: L input double; ref_colors output double; a input double; b input double; num_colors output double; Dist_Thresh input double
function [ref_colors, num_colors] = Segmentation(L,a,b,Dist_Thresh)
% This function tries segmentation by adding new reference colors everytime
% a pixel is found with a distance greater than a certain amount from
% every other reference color


[rows cols] = size(L);

Dist_Threshold = Dist_Thresh;% L = 0 to 100, a = -100 to 100, b = -100 to 100
                    % max dist = 300 -> 60/300 is 20%
x = 1;  % coefficients determining distance calculation
y = 1.5;
z = 1.5;

max_num_colors = 50;
ref_colors = zeros(max_num_colors,3);   % At most 50 different reference colors
LabelMatrix = zeros(rows,cols);
num_colors = 1;

center_row = floor(rows/2);
center_col = floor(cols/2);

% Define first reference color to be colr
ref_colors(1,:) = [L(center_row,center_col) a(center_row,center_col) b(center_row,center_col)];

flag = 0;
i = 1;
j = 1;
while(i <= rows)        % perform initial segmentation
    while(i <= rows && flag == 0)
        while(j <= cols && flag == 0)
            k = 1;
            min_dist = 1000;
            index = 1;
            while(k <= num_colors)
                
                % Loop through the list of stored colors, and find minimum
                % distance between ref_color(k,:) and [L(i,j), a(i,j), b(i,j)]
                dist = sqrt(x*(ref_colors(k,1) - L(i,j))^2 + y*(ref_colors(k,2) - a(i,j))^2 + z*(ref_colors(k,3) - b(i,j))^2);
                if(min_dist > dist)
                    min_dist = double(dist);
                    index = k;
                end
                k = k + 1;
            end
            if(j == 117)
                cow = 1;
            end
            if(min_dist > Dist_Threshold && num_colors < max_num_colors)
                ref_colors(num_colors+1,:) = [L(i,j) a(i,j) b(i,j)];
                num_colors = num_colors + 1;
                flag = 1;
                i = 0;
                j = 0;
                
            else
                LabelMatrix(i,j) = index;
            end
            j = j + 1;
        end
        j = 1;
        i = i + 1;
    end
    flag = 0;
end

% Go through image once more to get more accurate values for the different regions
ref_color_L_avg = zeros(50,1);
ref_color_a_avg = zeros(50,1);
ref_color_b_avg = zeros(50,1);
color_count = zeros(50,1);
for i = 1:rows
    for j = 1:cols
        index = LabelMatrix(i,j);
        ref_color_L_avg(index) = ref_color_L_avg(index) + L(i,j);
        ref_color_a_avg(index) = ref_color_a_avg(index) + a(i,j);
        ref_color_b_avg(index) = ref_color_b_avg(index) + b(i,j);
        color_count(index) = color_count(index) + 1;
    end
end
ref_color_L_avg = ref_color_L_avg ./ color_count;
ref_color_a_avg = ref_color_a_avg ./ color_count;
ref_color_b_avg = ref_color_b_avg ./ color_count;

for i = 1:num_colors
    ref_colors(i,1) = ref_color_L_avg(i);
    ref_colors(i,2) = ref_color_a_avg(i);
    ref_colors(i,3) = ref_color_b_avg(i);
end

return
